simulink model "c28069_DCcontrol_fbT"  (R2018b)
settings: Solver=ode4  StartTime=0.0  StopTime=inf  FixedStep=100e-6*0+0.0001  RelTol=1e-3
undefined symbols (not defined in the file or in its folder): serial
libraries: instrumentlib x2, powerlib_meascontrol x1
settings Model: Creator=matti  LastModifiedBy=matti
settings HardwareCC: ProdBitPerPointer=32  ProdBitPerSizeT=32  ProdBitPerPtrDiffT=32  ProdWordSize=32  ProdHWDeviceType=Intel->x86-32 (Windows32)
settings SFSimCC: SimUseLocalCustomCode=off
settings RTWCC: RTWUseLocalCustomCode=off
settings CodeAppCC: StateflowObjectComments=on
settings SimscapeCC: SimscapeNormalizeSystem=off

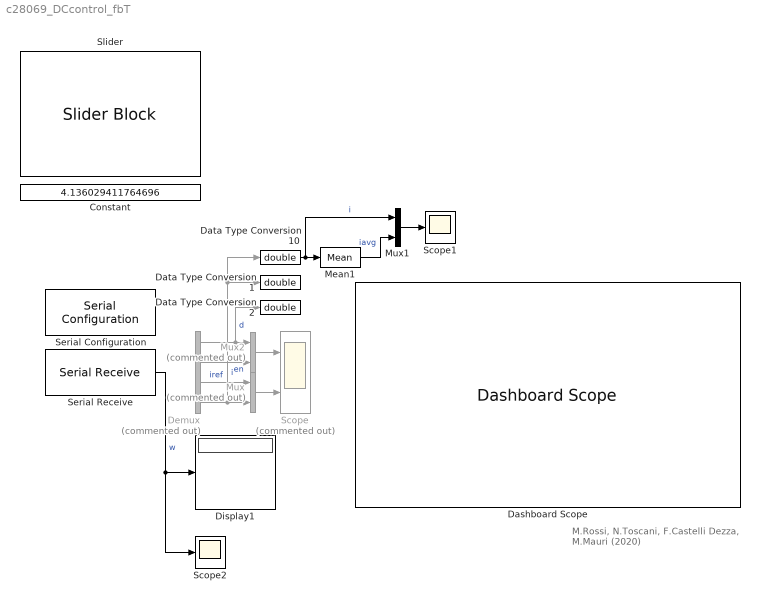
== system c28069_DCcontrol_fbT ==
  note: M.Rossi, N.Toscani, F.Castelli Dezza, M.Mauri (2020)
  Constant : Constant  Value=4.136029411764696  OutDataTypeStr=int16  SampleTime=.05
  Dashboard Scope : DashboardScope  WebBlockId=52  TimeSpan=30  Ymin=0  Ymax=2
  Data Type Conversion1 : DataTypeConversion  OutDataTypeStr=double
  Data Type Conversion10 : DataTypeConversion  OutDataTypeStr=double
  Data Type Conversion2 : DataTypeConversion  OutDataTypeStr=double
  Demux : Demux  Commented=on
  Display1 : Display
  Mean1 : powerlib_meascontrol/Measurements/Mean  Freq=20  Vinit=0  Ts=0.001
      settings: SourceProductName=Simscape Electrical
  Mux : Mux  Commented=on  Inputs=2
  Mux1 : Mux  Inputs=2
  Mux2 : Mux  Commented=on  Inputs=2
  Scope : Scope  Commented=on  NumInputPorts=2
  Scope1 : Scope
  Scope2 : Scope
  Serial Configuration : instrumentlib/Serial Configuration  Priority=-200000  ComPortMenu=<Please select a port...>  ComPort=COM20  ObjConstructor=serial('COM20');  BaudRate=115200  DataBits=8  Parity=none  StopBits=1  FlowControl=none  Timeout=10  ByteOrder=LittleEndian
  Serial Receive : instrumentlib/Serial Receive  ComPortMenu=<Please select a port...>  ComPort=COM20  ObjConstructor=serial('COM20');  Terminator=<none>  DataSize="[1  1]"  DataType=single  EnableBlockingMode=on  ActionDataUnavailable=Output last received value  CustomValue=0  SampleTime=0.01
  Slider : SliderBlock  WebBlockId=71  ScaleMin=-300  ScaleMax=300
  wires:
  Demux/3 -> Mux/1  "iref"
  Demux/1 -> Data Type Conversion2/1, Mux2/1  "d"
  Mean1/1 -> Mux1/2  "iavg"
  Data Type Conversion10/1 -> Mux1/1, Mean1/1  "i"
  ? -> Demux/1
  Mux/1 -> Scope/2
  Demux/4 -> Data Type Conversion10/1, Data Type Conversion1/1, Mux/2  "i"
  Mux2/1 -> Scope/1
  Demux/2 -> Mux2/2  "en"
  Mux1/1 -> Scope1/1
  Serial Receive/1 -> Display1/1, Scope2/1  "w"
